simulink model "state_estimators"  (R2025b)
settings: Solver=VariableStepAuto  StartTime=0.0  StopTime=10.0  RelTol=1e-3
libraries: battery x1, sharedTrackingLibrary x1
settings Model: Creator=Aditya  LastModifiedBy=jackpolloway

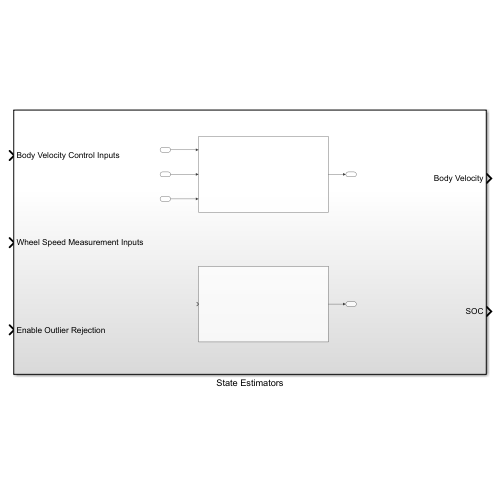
[thumbnail: Simulink's stored preview of the top-level diagram]
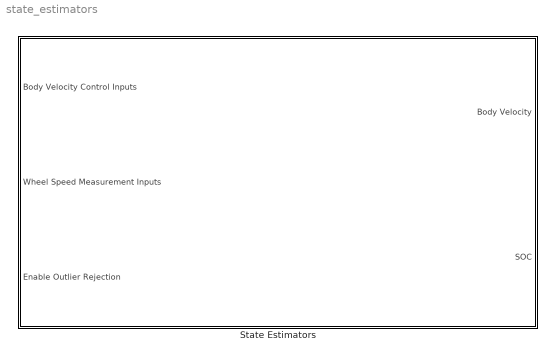
== system state_estimators ==
  State Estimators : Subsystem

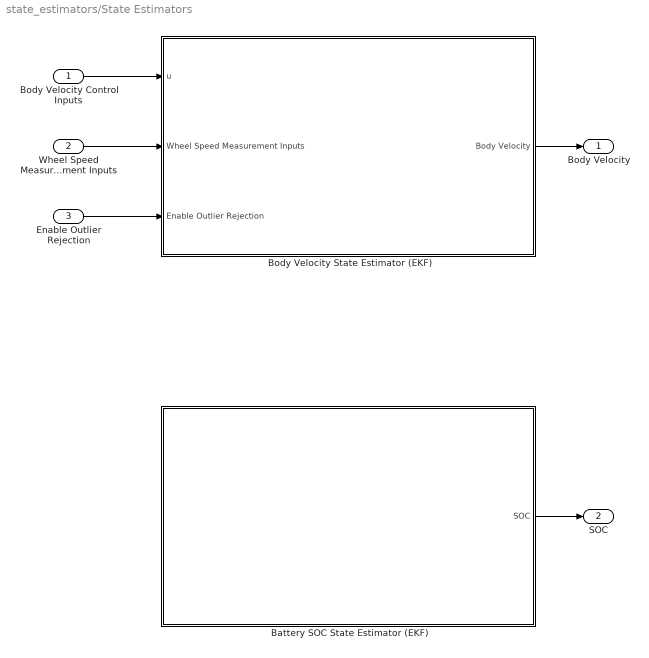
== system state_estimators/State Estimators ==
  Body Velocity Control Inputs : Inport
  Wheel Speed Measurement Inputs : Inport  Port=2
  Enable Outlier Rejection : Inport  Port=3
  Battery SOC State Estimator (EKF) : Subsystem
  Body Velocity State Estimator (EKF) : Subsystem
  Body Velocity : Outport
  SOC : Outport  Port=2
  wires:
  Body Velocity State Estimator (EKF)/1(Body Velocity) -> Body Velocity/1
  Battery SOC State Estimator (EKF)/1(SOC) -> SOC/1
  Body Velocity Control Inputs/1 -> Body Velocity State Estimator (EKF)/1(u)
  Wheel Speed Measurement Inputs/1 -> Body Velocity State Estimator (EKF)/2(Wheel Speed Measurement Inputs)
  Enable Outlier Rejection/1 -> Body Velocity State Estimator (EKF)/3(Enable Outlier Rejection)

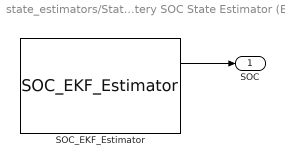
== system state_estimators/State Estimators/Battery SOC State Estimator (EKF) ==
  SOC_EKF_Estimator : battery/Subsystem/SOC_EKF_Estimator  SystemSampleTime=0.01  VariantActivationTime=update diagram  EmptyChoice=off  PassThrough=off  PassThroughVariantControl=(default)  EmptyChoiceVariantControl=(default)  AllowFlexibleInterface=on  Latency=0  AutoFrameSizeCalculation=off
  SOC : Outport
  wires:
  SOC_EKF_Estimator/1 -> SOC/1

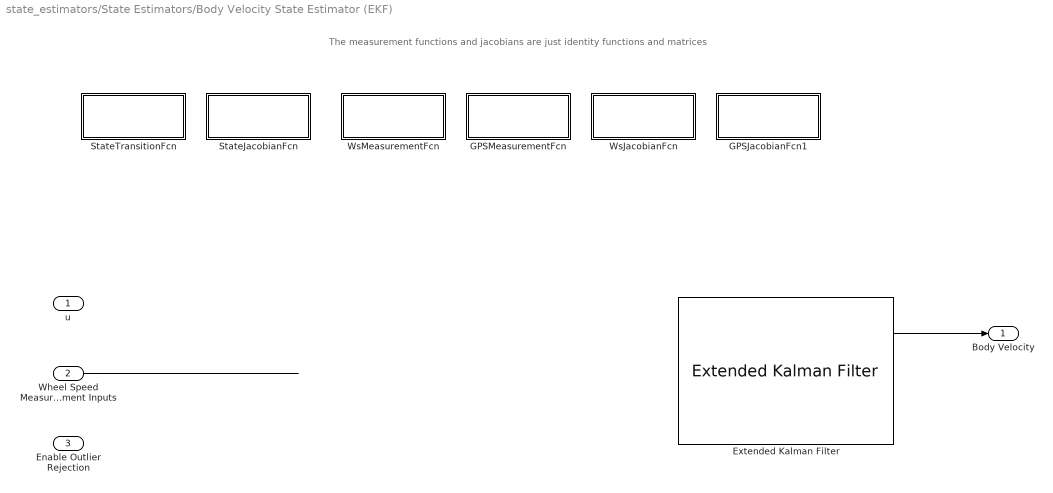
== system state_estimators/State Estimators/Body Velocity State Estimator (EKF) ==
  note: The measurement functions and jacobians are just identity functions and matrices
  u : Inport
  Wheel Speed Measurement Inputs : Inport  Port=2
  Enable Outlier Rejection : Inport  Port=3
  Extended Kalman Filter : sharedTrackingLibrary/Extended Kalman Filter  StateTransitionFcn=StateTransitionFcn  HasStateTransitionJacobianFcn=on  StateTransitionJacobianFcn=StateJacobianFcn  HasAdditiveProcessNoise=Nonadditive  ProcessNoise=1  HasTimeVaryingProcessNoise=off  HasStateTransitionFcnExtraArgument=0  InitialState=0  InitialStateCovariance=1  MeasurementFcn1=WsMeasurementFcn  HasMeasurementJacobianFcn1=on  MeasurementJacobianFcn1=WsJacobianFcn  HasMeasurementEnablePort1=on  HasAdditiveMeasurementNoise1=Nonadditive  MeasurementNoise1=1  HasTimeVaryingMeasurementNoise1=off  HasMeasurementFcnExtraArgument1=0  HasMeasurementWrapping1=off  MeasurementFcn2=GPSMeasurementFcn  HasMeasurementJacobianFcn2=on  MeasurementJacobianFcn2=GPSJacobianFcn  HasMeasurementEnablePort2=on  HasAdditiveMeasurementNoise2=Additive  MeasurementNoise2=1  HasTimeVaryingMeasurementNoise2=off  HasMeasurementFcnExtraArgument2=0  HasMeasurementWrapping2=off  MeasurementFcn3=myMeasurementFcn  HasMeasurementJacobianFcn3=off  HasMeasurementEnablePort3=off  HasAdditiveMeasurementNoise3=Additive  MeasurementNoise3=1  HasTimeVaryingMeasurementNoise3=off  HasMeasurementFcnExtraArgument3=0  HasMeasurementWrapping3=off  MeasurementFcn4=myMeasurementFcn  HasMeasurementJacobianFcn4=off  HasMeasurementEnablePort4=off  HasAdditiveMeasurementNoise4=Additive  MeasurementNoise4=1  HasTimeVaryingMeasurementNoise4=off  HasMeasurementFcnExtraArgument4=0  HasMeasurementWrapping4=off  MeasurementFcn5=myMeasurementFcn  HasMeasurementJacobianFcn5=off  HasMeasurementEnablePort5=off  HasAdditiveMeasurementNoise5=Additive  MeasurementNoise5=1  HasTimeVaryingMeasurementNoise5=off  HasMeasurementFcnExtraArgument5=0  HasMeasurementWrapping5=off  EnableMultirate=off  StateTransitionFcnSampleTime=1  MeasurementFcn1SampleTime=1  MeasurementFcn2SampleTime=1  MeasurementFcn3SampleTime=1  MeasurementFcn4SampleTime=1  MeasurementFcn5SampleTime=1  UseCurrentEstimator=on  OutputStateCovariance=on  DataType=double  SampleTime=1  NumberOfMeasurements=2
  GPSJacobianFcn1 : Subsystem  TreatAsAtomicUnit=on
  GPSMeasurementFcn : Subsystem  TreatAsAtomicUnit=on
  StateJacobianFcn : Subsystem  TreatAsAtomicUnit=on
  StateTransitionFcn : Subsystem  TreatAsAtomicUnit=on
  WsJacobianFcn : Subsystem  TreatAsAtomicUnit=on
  WsMeasurementFcn : Subsystem  TreatAsAtomicUnit=on
  Body Velocity : Outport
  wires:
  Wheel Speed Measurement Inputs/1 -> ?
  Extended Kalman Filter/1 -> Body Velocity/1

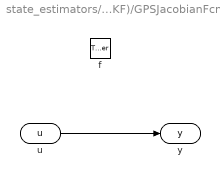
== system state_estimators/State Estimators/Body Velocity State Estimator (EKF)/GPSJacobianFcn1 ==
  f : TriggerPort  TriggerType=function-call  IsSimulinkFunction=on  FunctionName=f  FunctionVisibility=scoped  VariantControl=(inherit)
  u : ArgIn  DisableCoverage=on  ArgumentName=u
  y : ArgOut  DisableCoverage=on  ArgumentName=y
  wires:
  u/1 -> y/1

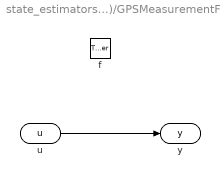
== system state_estimators/State Estimators/Body Velocity State Estimator (EKF)/GPSMeasurementFcn ==
  f : TriggerPort  TriggerType=function-call  IsSimulinkFunction=on  FunctionName=f  FunctionVisibility=scoped  VariantControl=(inherit)
  u : ArgIn  DisableCoverage=on  ArgumentName=u
  y : ArgOut  DisableCoverage=on  ArgumentName=y
  wires:
  u/1 -> y/1

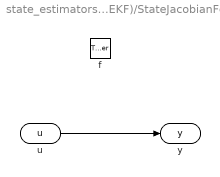
== system state_estimators/State Estimators/Body Velocity State Estimator (EKF)/StateJacobianFcn ==
  f : TriggerPort  TriggerType=function-call  IsSimulinkFunction=on  FunctionName=f  FunctionVisibility=scoped  VariantControl=(inherit)
  u : ArgIn  DisableCoverage=on  ArgumentName=u
  y : ArgOut  DisableCoverage=on  ArgumentName=y
  wires:
  u/1 -> y/1

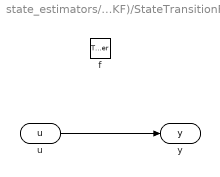
== system state_estimators/State Estimators/Body Velocity State Estimator (EKF)/StateTransitionFcn ==
  f : TriggerPort  TriggerType=function-call  IsSimulinkFunction=on  FunctionName=f  FunctionVisibility=scoped  VariantControl=(inherit)
  u : ArgIn  DisableCoverage=on  ArgumentName=u
  y : ArgOut  DisableCoverage=on  ArgumentName=y
  wires:
  u/1 -> y/1

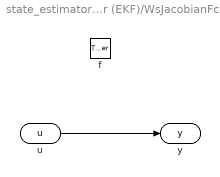
== system state_estimators/State Estimators/Body Velocity State Estimator (EKF)/WsJacobianFcn ==
  f : TriggerPort  TriggerType=function-call  IsSimulinkFunction=on  FunctionName=f  FunctionVisibility=scoped  VariantControl=(inherit)
  u : ArgIn  DisableCoverage=on  ArgumentName=u
  y : ArgOut  DisableCoverage=on  ArgumentName=y
  wires:
  u/1 -> y/1

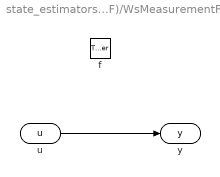
== system state_estimators/State Estimators/Body Velocity State Estimator (EKF)/WsMeasurementFcn ==
  f : TriggerPort  TriggerType=function-call  IsSimulinkFunction=on  FunctionName=f  FunctionVisibility=scoped  VariantControl=(inherit)
  u : ArgIn  DisableCoverage=on  ArgumentName=u
  y : ArgOut  DisableCoverage=on  ArgumentName=y
  wires:
  u/1 -> y/1
